simulink model "Tank_level_control_BF_equation_model_TZ_DDT"  (R2022a)
settings: Solver=FixedStepAuto  StartTime=0.0  StopTime=1000  FixedStep=0.1  RelTol=1e-3
settings Model: Creator=dtheilli  LastModifiedBy=julie
settings DebuggingCC: UnconnectedInputMsg=warning  UnconnectedOutputMsg=warning  UnconnectedLineMsg=warning
settings RTWCC: DLArmComputeVersion=19.05

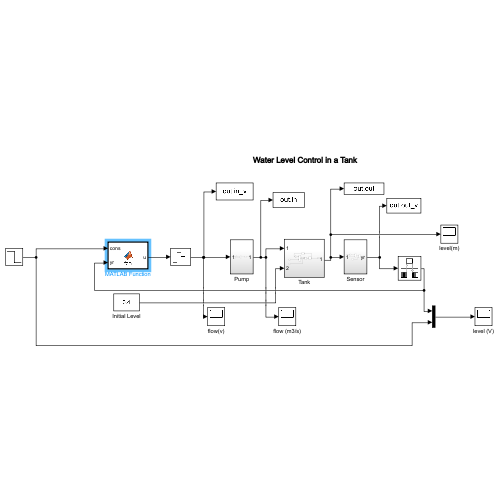
[thumbnail: Simulink's stored preview of the top-level diagram]
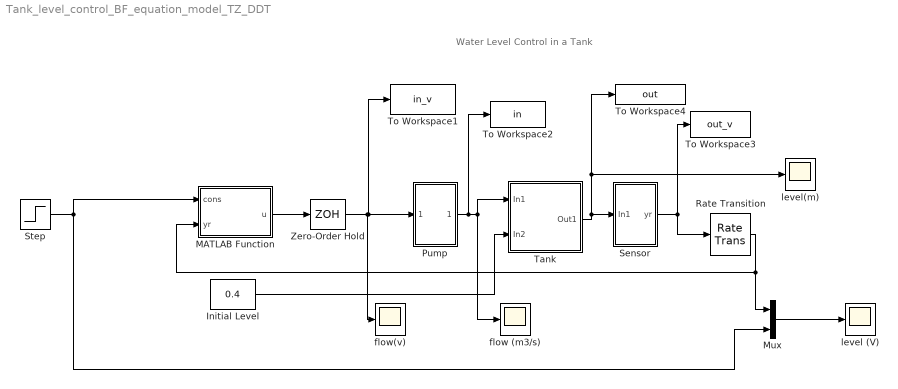
== system Tank_level_control_BF_equation_model_TZ_DDT ==
  note: Water Level Control in a Tank
  Initial Level : Constant  Value=0.4
  MATLAB Function : MATLAB Function  TreatAsAtomicUnit=on
  Mux : Mux  Inputs=2
  Pump : Subsystem
  Rate Transition : RateTransition  OutPortSampleTime=1
  Sensor : Subsystem
  Step : Step  Time=500  Before=-27.9242*0.4+9.0480  After=-27.9242*0.45+9.0480  SampleTime=0
  Tank : Subsystem
  To Workspace1 : ToWorkspace  VariableName=in_v  SaveFormat=Timeseries  SampleTime=-1
  To Workspace2 : ToWorkspace  VariableName=in  SaveFormat=Timeseries  SampleTime=-1
  To Workspace3 : ToWorkspace  VariableName=out_v  SaveFormat=Timeseries  SampleTime=-1
  To Workspace4 : ToWorkspace  VariableName=out  SaveFormat=Timeseries  SampleTime=-1
  Zero-Order Hold : ZeroOrderHold  SampleTime=10
  flow (m3/s) : Scope
  flow(v) : Scope
  level (V) : Scope
  level(m) : Scope
  wires:
  Tank/1(Out1) -> To Workspace4/1, level(m)/1, Sensor/1(In1)
  Pump/1(Out1) -> Tank/1(In1), flow (m3/s)/1, To Workspace2/1
  Sensor/1(yr) -> Rate Transition/1, To Workspace3/1
  Initial Level/1 -> Tank/2(In2)
  Mux/1 -> level (V)/1
  Zero-Order Hold/1 -> flow(v)/1, Pump/1(In1), To Workspace1/1
  Step/1 -> Mux/2, MATLAB Function/1(cons)
  MATLAB Function/1(u) -> Zero-Order Hold/1
  Rate Transition/1 -> MATLAB Function/2(yr), Mux/1

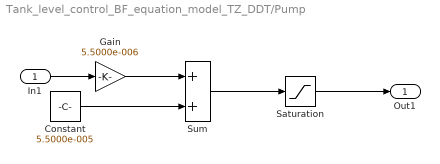
== system Tank_level_control_BF_equation_model_TZ_DDT/Pump ==
  In1 : Inport
  Constant : Constant  Value=5.5000e-005
  Gain : Gain  Gain=5.5000e-006
  Saturation : Saturate  UpperLimit=1.1e-4  LowerLimit=0
  Sum : Sum
  Out1 : Outport
  wires:
  In1/1 -> Gain/1
  Gain/1 -> Sum/1
  Constant/1 -> Sum/2
  Saturation/1 -> Out1/1
  Sum/1 -> Saturation/1

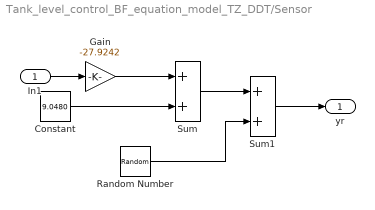
== system Tank_level_control_BF_equation_model_TZ_DDT/Sensor ==
  In1 : Inport
  Constant : Constant  Value=9.0480
  Gain : Gain  Gain=-27.9242
  Random Number : RandomNumber  Variance=0.00005  SampleTime=0.1
  Sum : Sum
  Sum1 : Sum
  yr : Outport
  wires:
  In1/1 -> Gain/1
  Gain/1 -> Sum/1
  Constant/1 -> Sum/2
  Sum/1 -> Sum1/1
  Sum1/1 -> yr/1
  Random Number/1 -> Sum1/2

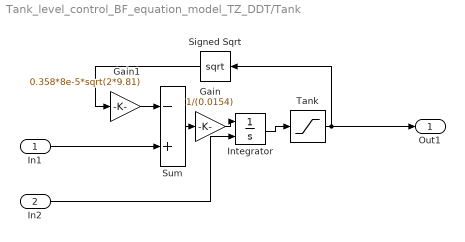
== system Tank_level_control_BF_equation_model_TZ_DDT/Tank ==
  In1 : Inport
  In2 : Inport  Port=2
  Gain : Gain  Gain=1/(0.0154)  SaturateOnIntegerOverflow=on  OutDataTypeStr=Inherit: Same as input  ParamDataTypeStr=Inherit: Same as input
  Gain1 : Gain  Gain=0.358*8e-5*sqrt(2*9.81)  SaturateOnIntegerOverflow=on  OutDataTypeStr=Inherit: Same as input  ParamDataTypeStr=Inherit: Same as input
  Integrator : Integrator  InitialConditionSource=external  InitialCondition=0.4
  Signed Sqrt : Sqrt
  Sum : Sum  Inputs=-+  InputSameDT=on  SaturateOnIntegerOverflow=on  OutDataTypeStr=Inherit: Same as first input
  Tank : Saturate  UpperLimit=0.6  LowerLimit=0
  Out1 : Outport
  wires:
  In1/1 -> Sum/2
  Gain1/1 -> Sum/1
  Sum/1 -> Gain/1
  Tank/1 -> Signed Sqrt/1, Out1/1
  Signed Sqrt/1 -> Gain1/1
  Integrator/1 -> Tank/1
  Gain/1 -> Integrator/1
  In2/1 -> Integrator/2

== matlab function Tank_level_control_BF_equation_model_TZ_DDT/MATLAB Function ==
  data: cons input; u output; yr input
function u = fcn(cons,yr)

u=13*(yr-cons) + integral(yr,0,inf);
